simulink model "Simscape2"  (R2025b)
settings: Solver=FixedStepAuto  StartTime=0.0  StopTime=tend  FixedStep=TT_c  RelTol=1e-4  EnableMultiTasking=on
values from neighbouring files (symbols this model uses):
  alpha = 3.93e-3    (= 0.00393)    [Script_caricamento_dati_simscape2.m]
  Cr = In*2/4*Kc_act    (= 0.548435475)    [Script_caricamento_dati_simscape2.m]
  Crn = In*Kc_nom    (= 1.09116)    [Script_caricamento_dati_simscape2.m]
  f_AC_corr = [f_AC(1); f_AC(5:end)]    [Script_caricamento_dati_simscape2.m]
  In = 14    [Script_caricamento_dati_simscape2.m]
  isq0 = (B*wdq0/J + np*Cr0/J)/(Kc*np/J + ms*np^(2)*(Lsd-Lsq)*isd0/(2*J))    (= 0)    [Script_caricamento_dati_simscape2.m]
  J = 0.04e-3*3    (= 0.00012)    [Script_caricamento_dati_simscape2.m]
  kaisd = 1000    [Script_caricamento_dati_simscape2.m]
  kaisq = 1000    [Script_caricamento_dati_simscape2.m]
  kawr = 1000    [Script_caricamento_dati_simscape2.m]
  kiisd = kpisd/tiisd    (= 13158.2733813)    [Script_caricamento_dati_simscape2.m]
  kiisq = kpisq/tiisq    (= 13158.2733813)    [Script_caricamento_dati_simscape2.m]
  kiPLL = 2.5e6    (= 2500000)    [Script_caricamento_dati_simscape2.m]
  kiwr = 600    [Script_caricamento_dati_simscape2.m]
  kpisd = 23.6    [Script_caricamento_dati_simscape2.m]
  kpisq = 23.6    [Script_caricamento_dati_simscape2.m]
  kpPLL = 15    [Script_caricamento_dati_simscape2.m]
  kpwr = 0.12    [Script_caricamento_dati_simscape2.m]
  lambdam_Matrix = [1 1 1; 1 1 1; 1 1 1]    [Script_caricamento_dati_simscape2.m]
  Lsd = 1.251e-3    (= 0.001251)    [Script_caricamento_dati_simscape2.m]
  Lsd_Matrix = [1 1 1; 1 1 1; 1 1 1]    [Script_caricamento_dati_simscape2.m]
  Lsq = Lsd    (= 0.001251)    [Script_caricamento_dati_simscape2.m]
  Lsq_Matrix = [1 1 1; 1 1 1; 1 1 1]    [Script_caricamento_dati_simscape2.m]
  np = 2    [Script_caricamento_dati_simscape2.m]
  np_res = 2    [Script_caricamento_dati_simscape2.m]
  Pmax = 3*Vdc/2*Imax    (= 17010)    [Script_caricamento_dati_simscape2.m]
  Psim = 26.82e-3    (= 0.02682)    [Script_caricamento_dati_simscape2.m]
  Ratio_Rs_AC = (Rs_AC_corr-Rs)/Rs    [Script_caricamento_dati_simscape2.m]
  Rs = 0.6975    [Script_caricamento_dati_simscape2.m]
  Tmax = 1.5*Crn    (= 1.63674)    [Script_caricamento_dati_simscape2.m]
  Tphase = 100    [Script_caricamento_dati_simscape2.m]
  Trif = 298.15    [Script_caricamento_dati_simscape2.m]
  TT_c = TT_swt/100    (= 5e-07)    [Script_caricamento_dati_simscape2.m]
  TT_sc = 5e-5    (= 5e-05)    [Script_caricamento_dati_simscape2.m]
  TT_swt = 5e-5    (= 5e-05)    [Script_caricamento_dati_simscape2.m]
  Vdc = 540    [Script_caricamento_dati_simscape2.m]
  wrn = 30000    [Script_caricamento_dati_simscape2.m]
  wrr = wrn/5*1    (= 6000)    [Script_caricamento_dati_simscape2.m]
undefined symbols (not defined in the file or in its folder): denZC_id, denZC_iq, ee_sli_rtmsupport, gcbh, lambdam, numZC_id, numZC_iq
libraries: fl_lib x28, nesl_utility x22, ee_lib x14, eeTransforms x7, eeGeneralControl x6, eeDiscretePi x2, dspstat3 x1, batteryecm_lib x1, eeDqVoltageLimiter x1, eePmsmCurrentReferenceGen x1, eeVelocityController x1, eePwmGeneratorTwoLevel x1
(part 3 of 3)

== system Simscape2/PMSM Field-Oriented Control/Inner loop control ==
  idq_ref : Inport
  wElectrical : Inport  Port=2
  iabc : Inport  Port=3
  theta : Inport  Port=4
  Vdc : Inport  Port=5
  Constant : Constant  Value=0  SampleTime=-1
  Gain : Gain  Gain=1/sqrt(3)
  PMSM Current Controller with Pre-Control : Subsystem  AncestorBlock=eePmsmCurrentController/PMSM Current Controller with Pre-Control  LoadFcn=ee_sli_rtmsupport( 'loadfcn', gcbh );  mask(PMSM Current Controller with Pre-Control){Kp_id=Kp_id, Ki_id=Ki_id, Kaw_id=Kaw_id, Kp_iq=Kp_iq, Ki_iq=Ki_iq, Kaw_iq=Kaw_iq, Ts=Tsc, Tsd=0.001, AxisPrio=D-Q equivalence, ActZC=off, ActFF=on, idVect=idVect, iqVect=iqVect, LdMatrix=LdMatrix, LqMatrix=LqMatrix, psimMatrix=psimMatrix}
      mask prompts: Kp_id "physmod:ee:library:comments:control:eePmsmCurrentController:DaxisCurrentProportionalGain_MP"; Ki_id "physmod:ee:library:comments:control:eePmsmCurrentController:DaxisCurrentIntegralGain_MP"; Kaw_id "physmod:ee:library:comments:control:eePmsmCurrentController:DaxisCurrentAntiwindupGain_MP"; Kp_iq "physmod:ee:library:comments:control:eePmsmCurrentController:QaxisCurrentProportionalGain_MP"; Ki_iq "physmod:ee:library:comments:control:eePmsmCurrentController:QaxisCurrentIntegralGain_MP"; Kaw_iq "physmod:ee:library:comments:control:eePmsmCurrentController:QaxisCurrentAntiwindupGain_MP"; Ts "physmod:ee:library:comments:control:eePmsmCurrentController:SampleTime1ForInherited_MP"; Tsd "physmod:ee:library:comments:control:eePmsmCurrentController:DiscretizationSampleTime_MP"; AxisPrio "physmod:ee:library:comments:control:eePmsmCurrentController:AxisPrioritization_MP"; ActZC "physmod:ee:library:comments:control:eePmsmCurrentController:EnableZeroCancellation_MP"; ActFF "physmod:ee:library:comments:control:eePmsmCurrentController:EnablePrecontrolVoltage_MP"; idVect "physmod:ee:library:comments:control:eePmsmCurrentController:DaxisCurrentVectorIdA_MP"; iqVect "physmod:ee:library:comments:control:eePmsmCurrentController:QaxisCurrentVectorIqA_MP"; LdMatrix "physmod:ee:library:comments:control:eePmsmCurrentController:LdMatrixLdidiqH_MP"; LqMatrix "physmod:ee:library:comments:control:eePmsmCurrentController:LqMatrixLqidiqH_MP"; psimMatrix "physmod:ee:library:comments:control:eePmsmCurrentController:PermanentMagnetFluxLinkageMatrixPMidiqWb_MP"
      mask help: physmod:ee:library:comments:control:eePmsmCurrentController:PMSMCurrentControllerWithPreControl_MD
      mask init:
      | [Tsd, numZC_id, denZC_id, numZC_iq, denZC_iq] = ee.mask.initializePmsmCurrentController(ActZC,Ts,Tsd,Kp_id,Ki_id,Kp_iq,Ki_iq);
      | 
      | if length(idVect) < 2            
      | 	error(message('physmod:simscape:compiler:patterns:checks:LengthGreaterThanOrEqual',getString(message('physmod:ee:library:comments:control:eePmsmCurrentController:DaxisCurrentVectorIdA_MP')), '2'));            
      | end
      | if ~all(diff(idVect) > 0)            
      | 	error(message('physmod:simscape:compiler:patterns:checks:StrictlyAscendingVec',getString(message('physmod:ee:library:comments:control:eePmsmCurrentController:DaxisCurrentVectorIdA_MP'))));            
      | end
      | if length(iqVect) < 2            
      | 	error(message('physmod:simscape:compiler:patterns:checks:LengthGreaterThanOrEqual',getString(message('physmod:ee:library:comments:control:eePmsmCurrentController:QaxisCurrentVectorIqA_MP')), '2'));            
      | end
      | if ~all(diff(iqVect) > 0)            
      | 	error(message('physmod:simscape:compiler:patterns:checks:StrictlyAscendingVec',getString(message('physmod:ee:library:comments:control:eePmsmCurrentController:QaxisCurrentVectorIqA_MP'))));            
      | end
      | if ~all(size(LdMatrix) == [length(idVect), length(iqVect)])            
      | 	error(message('physmod:simscape:compiler:patterns:checks:Size2DEqual',getString(message('physmod:ee:library:comments:control:eePmsmCurrentController:LdMatrixLdidiqH_MP')), getString(message('physmod:ee:library:comments:control:eePmsmCurrentController:DaxisCurrentVectorIdA_MP')), getString(message('physmod:ee:library:comments:control:eePmsmCurrentController:QaxisCurrentVectorIqA_MP'))));            
      | end
      | if ~all(size(LqMatrix) == [length(idVect), length(iqVect)])            
      | 	error(message('physmod:simscape:compiler:patterns:checks:Size2DEqual',getString(message('physmod:ee:library:comments:control:eePmsmCurrentController:LqMatrixLqidiqH_MP')), getString(message('physmod:ee:library:comments:control:eePmsmCurrentController:DaxisCurrentVectorIdA_MP')), getString(message('physmod:ee:library:comments:control:eePmsmCurrentController:QaxisCurrentVectorIqA_MP'))));            
      | end
      | if ~all(size(psimMatrix) == [length(idVect), length(iqVect)])            
      | 	error(message('physmod:simscape:compiler:patterns:checks:Size2DEqual',getString(message('physmod:ee:library:comments:control:eePmsmCurrentController:PermanentMagnetFluxLinkageMatrixPMidiqWb_MP')), getString(message('physmod:ee:library:comments:control:eePmsmCurrentController:DaxisCurrentVectorIdA_MP')), getString(message('physmod:ee:library:comments:control:eePmsmCurrentController:QaxisCurrentVectorIqA_MP'))));            
      | end
      settings: CopyFcn=ee_sli_rtmsupport( 'copyfcn', gcbh );  DeleteFcn=ee_sli_rtmsupport( 'deletefcn', gcbh );  ModelCloseFcn=ee_sli_rtmsupport( 'modelclosefcn', gcbh );  PostSaveFcn=ee_sli_rtmsupport( 'postsavefcn', gcbh );  PreCopyFcn=ee_sli_rtmsupport( 'precopyfcn', gcbh );  OpenFcn=ee_sli_rtmsupport( 'openfcn', gcbh );  CloseFcn=ee_sli_rtmsupport( 'closefcn', gcbh );  PreDeleteFcn=ee_sli_rtmsupport( 'predeletefcn', gcbh );
      mask Help: web(nesl_help(gcbh))
      mask Callback Ts: ee.mask.callbackZeroCancellation(gcb);
      mask TypeOptions AxisPrio: d-q Voltage Limiter/AxisPrio
      mask Callback ActZC: ee.mask.callbackZeroCancellation(gcb);
      mask DialogControl Container3 Prompt: physmod:ee:library:comments:control:eePmsmCurrentController:tab_ControlParameters
      mask DialogControl Kp_id Prompt: D-axis current proportional gain
      mask DialogControl Ki_id Prompt: D-axis current integral gain
      mask DialogControl Kaw_id Prompt: D-axis current anti-windup gain
      mask DialogControl Kp_iq Prompt: Q-axis current proportional gain
      mask DialogControl Ki_iq Prompt: Q-axis current integral gain
      mask DialogControl Kaw_iq Prompt: Q-axis current anti-windup gain
      mask DialogControl Ts Prompt: Sample time (-1 for inherited)
      mask DialogControl Tsd Prompt: Discretization sample time
      mask DialogControl AxisPrio Prompt: Axis prioritization
      mask DialogControl ActZC Prompt: Enable zero cancellation
      mask DialogControl ActFF Prompt: Enable pre-control voltage
      mask DialogControl Container4 Prompt: physmod:ee:library:comments:control:eePmsmCurrentController:tab_PreControlParameters
      mask DialogControl idVect Prompt: D-axis current vector, id (A)
      mask DialogControl iqVect Prompt: Q-axis current vector, iq (A)
      mask DialogControl LdMatrix Prompt: Ld matrix, Ld(id,iq), (H)
      mask DialogControl LqMatrix Prompt: Lq matrix, Lq(id,iq), (H)
      mask DialogControl psimMatrix Prompt: Permanent magnet flux linkage matrix, PM(id,iq), (Wb)
  Park Transform : eeTransforms/Park Transform  AxisAlignment=D-axis  PowerInvariant=off
  Selector : Selector  InputPortWidth=3  IndexOptions=Index vector (dialog)  Indices=[1 2]  OutputSizes=1
  vdqRef : Outport  VectorParamsAs1DForOutWhenUnconnected=off
  idq : Outport  Port=2  VectorParamsAs1DForOutWhenUnconnected=off
  wires:
  PMSM Current Controller with Pre-Control/1(vdqRef) -> vdqRef/1
  Vdc/1 -> Gain/1
  wElectrical/1 -> PMSM Current Controller with Pre-Control/3(wElectrical)
  theta/1 -> Park Transform/2
  iabc/1 -> Park Transform/1
  idq_ref/1 -> PMSM Current Controller with Pre-Control/1(idqRef)
  Park Transform/1 -> Selector/1
  Gain/1 -> PMSM Current Controller with Pre-Control/4(VphMax)
  Selector/1 -> idq/1, PMSM Current Controller with Pre-Control/2(idq)
  Constant/1 -> PMSM Current Controller with Pre-Control/5(Reset)

== system Simscape2/PMSM Field-Oriented Control/Input interface ==
  iabcSens : Inport
  wSens : Inport  Port=2
  thSens : Inport  Port=3
  VdcSens : Inport  Port=4
  2*pi : Constant  Value=2*pi  SampleTime=Tsc
  Math Function : Math  Operator=mod  SignedPower=on
  Relay : Relay  OnSwitchValue=Vdc_on  OffSwitchValue=0.5*Vdc_on
  pole pairs : Gain  Gain=p
  "pole pairs " : Gain  Gain=p
  wElectrical : Outport  VectorParamsAs1DForOutWhenUnconnected=off
  iabc : Outport  Port=2  VectorParamsAs1DForOutWhenUnconnected=off
  theta : Outport  Port=3  VectorParamsAs1DForOutWhenUnconnected=off
  Vdc : Outport  Port=4  VectorParamsAs1DForOutWhenUnconnected=off
  PwmEnable : Outport  Port=5  VectorParamsAs1DForOutWhenUnconnected=off
  wires:
  VdcSens/1 -> Vdc/1, Relay/1
  Relay/1 -> PwmEnable/1
  Math Function/1 -> theta/1
  2*pi/1 -> Math Function/2
  "pole pairs "/1 -> Math Function/1
  iabcSens/1 -> iabc/1
  wSens/1 -> pole pairs/1
  thSens/1 -> "pole pairs "/1
  pole pairs/1 -> wElectrical/1

== system Simscape2/PMSM Field-Oriented Control/Outer loop control ==
  Reference : Inport
  wElectrical : Inport  Port=2
  Vdc : Inport  Port=3
  Constant : Constant  Value=0  SampleTime=-1
  PMSM Current Reference Generator : eePmsmCurrentReferenceGen/PMSM Current Reference Generator  Vnom=Vnom  Pmax=Pmax  Tmax=Tmax  Ts=Tsc  RefType=Zero d-axis control  rpmVec=rpmVec  TqVec=TqVec  VdcVec=VdcVec  PWMMode=SPWM: sinusoidal PWM  ModFactor=ModFactor  idMatrix=idMatrix  iqMatrix=iqMatrix  p=p  psim=psim  Ld=Ld  Lq=Lq  Rs=Rs  RefExpEnable=0
      link override idRef: Value=0
  Tq Selector : Subsystem
  Velocity Controller : eeVelocityController/Velocity Controller  CtrlType=PI control  Kp_w=Kp_w  Ki_w=Ki_w  Kv_w=Kv_w  Kaw_w=Kaw_w  Ts=Tsc  Tsd=0.001  ActZC=off
  elec->mech : Gain  Gain=1/p
  idqRef : Outport  VectorParamsAs1DForOutWhenUnconnected=off
  TqRef : Outport  Port=2  VectorParamsAs1DForOutWhenUnconnected=off
  TqLim : Outport  Port=3  VectorParamsAs1DForOutWhenUnconnected=off
  wires:
  Velocity Controller/1 -> Tq Selector/2(TqRefUnsat)
  Tq Selector/1(TqRef) -> PMSM Current Reference Generator/1
  Constant/1 -> Velocity Controller/4
  elec->mech/1 -> Velocity Controller/2, PMSM Current Reference Generator/2
  PMSM Current Reference Generator/3 -> TqLim/1
  PMSM Current Reference Generator/2 -> TqRef/1, Velocity Controller/3
  PMSM Current Reference Generator/1 -> idqRef/1
  Vdc/1 -> PMSM Current Reference Generator/3
  wElectrical/1 -> elec->mech/1
  Reference/1 -> Tq Selector/1(Reference), Velocity Controller/1

== system Simscape2/PMSM Field-Oriented Control/PWM ==
  vdqRef : Inport
  theta : Inport  Port=2
  Vdc : Inport  Port=3
  PwmEnable : Inport  Port=4
  Constant : Constant  Value=0  SampleTime=Tsc
  Inverse Park Transform : eeTransforms/Inverse Park Transform  AxisAlignment=D-axis  PowerInvariant=off
  Mux : Mux  Inputs=2
  "PWM Generator (Three-phase, Two-level)" : eePwmGeneratorTwoLevel/PWM Generator (Three-phase, Two-level)  PWMMode=Continuous PWM (CPWM)  CPWMMode=SPWM: sinusoidal PWM  DPWMMode=60 DPWM: 60 degree discontinuous PWM  fsw=fsw  Ts=Ts
      settings: SamplingMode=Symmetric
  Switch1 : Switch  Criteria=u2 > Threshold  SaturateOnIntegerOverflow=off  InputSameDT=off
  To Workspace : ToWorkspace  VariableName=Vabc_ref  SampleTime=-1
  Unit Delay2 : UnitDelay  SampleTime=Tsc  HasFrameUpgradeWarning=on
  Zero vector : Constant  Value=zeros(6,1)  SampleTime=Ts
  G : Outport  VectorParamsAs1DForOutWhenUnconnected=off
  ModWave : Outport  Port=2  SampleTime=Tsc  VectorParamsAs1DForOutWhenUnconnected=off
  wires:
  Unit Delay2/1 -> Switch1/2
  Vdc/1 -> "PWM Generator (Three-phase, Two-level)"/2
  Inverse Park Transform/1 -> To Workspace/1, "PWM Generator (Three-phase, Two-level)"/1
  Switch1/1 -> G/1
  Zero vector/1 -> Switch1/3
  PwmEnable/1 -> Unit Delay2/1
  "PWM Generator (Three-phase, Two-level)"/1 -> Switch1/1
  "PWM Generator (Three-phase, Two-level)"/2 -> ModWave/1
  Constant/1 -> Mux/2
  Mux/1 -> Inverse Park Transform/1
  vdqRef/1 -> Mux/1
  theta/1 -> Inverse Park Transform/2

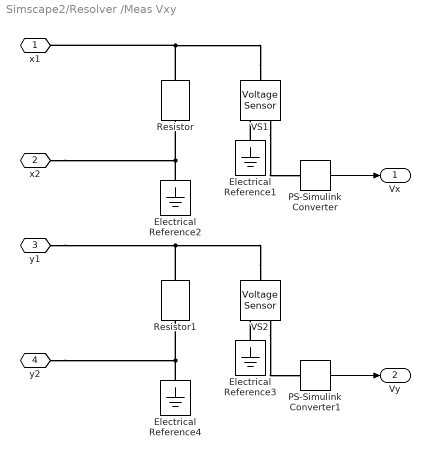
== system Simscape2/Resolver /Meas Vxy ==
  Electrical Reference{1..4} (4 alike) : fl_lib/Electrical/Electrical Elements/Electrical Reference
  PS-Simulink Converter : nesl_utility/PS-Simulink Converter  PhysicalDomain=network_engine_domain  SubClassName=ps_output  LeftPortType=input  RightPortType=output  PseudoPeriodic=off  Frequencies=[]  Unit=1  AffineConversion=off
  PS-Simulink Converter1 : nesl_utility/PS-Simulink Converter  PhysicalDomain=network_engine_domain  SubClassName=ps_output  LeftPortType=input  RightPortType=output  PseudoPeriodic=off  Frequencies=[]  Unit=1  AffineConversion=off
  Resistor : fl_lib/Electrical/Electrical Elements/Resistor  R=1e3 Ohm  i_specify=off  i_priority=None  i=0 A  i_nominal_specify=off  i_nominal_unit=A  i_nominal_value=1  v_specify=off  v_priority=None  v=0 V  v_nominal_specify=off  v_nominal_unit=V  v_nominal_value=1
  Resistor1 : fl_lib/Electrical/Electrical Elements/Resistor  R=1e3 Ohm  i_specify=off  i_priority=None  i=0 A  i_nominal_specify=off  i_nominal_unit=A  i_nominal_value=1  v_specify=off  v_priority=None  v=0 V  v_nominal_specify=off  v_nominal_unit=V  v_nominal_value=1
  VS1 : fl_lib/Electrical/Electrical Sensors/Voltage Sensor
  VS2 : fl_lib/Electrical/Electrical Sensors/Voltage Sensor
  x1 : PMIOPort  Side=Left
  x2 : PMIOPort  Port=2  Side=Left
  y1 : PMIOPort  Port=3  Side=Left
  y2 : PMIOPort  Port=4  Side=Left
  Vx : Outport
  Vy : Outport  Port=2
  wires:
  PS-Simulink Converter/1 -> Vx/1
  PS-Simulink Converter1/1 -> Vy/1
  connections:
  VS1/LConn1 -- x1/RConn1 -- Resistor/LConn1
  VS1/RConn1 -- PS-Simulink Converter/LConn1
  Resistor/RConn1 -- x2/RConn1 -- Electrical Reference2/LConn1
  Electrical Reference1/LConn1 -- VS1/RConn2
  y2/RConn1 -- Electrical Reference4/LConn1 -- Resistor1/RConn1
  VS2/LConn1 -- y1/RConn1 -- Resistor1/LConn1
  Electrical Reference3/LConn1 -- VS2/RConn2
  VS2/RConn1 -- PS-Simulink Converter1/LConn1

== system Simscape2/Resolver /Vp ==
  Electrical Reference1 : fl_lib/Electrical/Electrical Elements/Electrical Reference
  PS-Simulink Converter2 : nesl_utility/PS-Simulink Converter  PhysicalDomain=network_engine_domain  SubClassName=ps_output  LeftPortType=input  RightPortType=output  PseudoPeriodic=off  Frequencies=[]  Unit=1  AffineConversion=off
  VS1 : fl_lib/Electrical/Electrical Sensors/Voltage Sensor
  Vp1 : fl_lib/Electrical/Electrical Sources/AC Voltage Source  amp=5 V  shift=0 rad  frequency=1e4 Hz  omega=0 rad/s
  p1 : PMIOPort  Side=Right
  p2 : PMIOPort  Port=2  Side=Right
  Vp : Outport
  wires:
  PS-Simulink Converter2/1 -> Vp/1
  connections:
  VS1/RConn1 -- PS-Simulink Converter2/LConn1
  Electrical Reference1/LConn1 -- p2/RConn1 -- VS1/RConn2 -- Vp1/RConn1
  VS1/LConn1 -- Vp1/LConn1 -- p1/RConn1

== system Simscape2/Sensing currents1/LEM current sensor uncertainty ==
  In1 : Inport
  Demux : Demux  Outputs=3
  Mux : Mux  Inputs=3
  Offset : Constant  Value=0
  Offset1 : Constant  Value=0
  Offset2 : Constant  Value=0
  Product : Product
  Product2 : Product
  Product3 : Product
  Sum : Sum  Inputs=|++
  Sum1 : Sum  Inputs=|++
  Sum2 : Sum  Inputs=|++
  Uniform Random Number : UniformRandomNumber  Minimum=-0.0065  Maximum=0.0065  SampleTime=TT_c
  Out1 : Outport
  wires:
  Product/1 -> Sum/2
  Sum1/1 -> Mux/2
  Uniform Random Number/1 -> Product3/2, Product2/2, Product/2
  In1/1 -> Demux/1
  Offset/1 -> Sum/1
  Sum2/1 -> Mux/3
  Sum/1 -> Mux/1
  Mux/1 -> Out1/1
  Demux/1 -> Product/1
  Product3/1 -> Sum2/2
  Product2/1 -> Sum1/2
  Demux/3 -> Product3/1
  Demux/2 -> Product2/1
  Offset1/1 -> Sum1/1
  Offset2/1 -> Sum2/1

== system Simscape2/Three-phase inverter/LEM voltage sensor uncertainty ==
  In1 : Inport
  Product : Product
  Uniform Random Number : UniformRandomNumber  Minimum=-0.008  Maximum=0.008  SampleTime=TT_c
  Out1 : Outport
  wires:
  Uniform Random Number/1 -> Product/2
  In1/1 -> Product/1
  Product/1 -> Out1/1

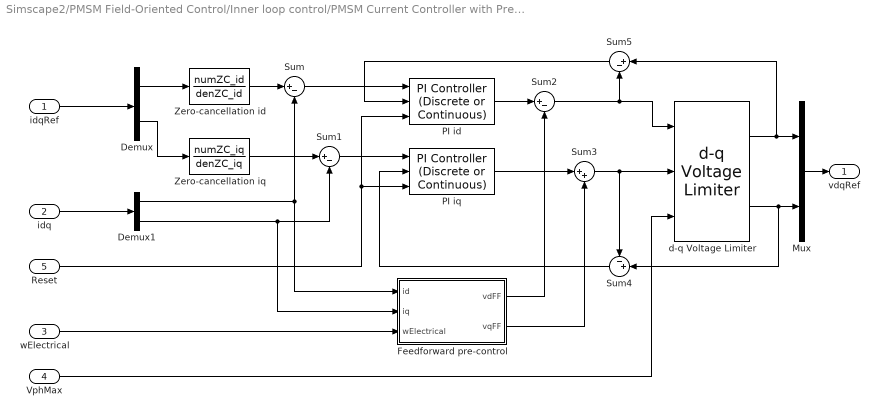
== system Simscape2/PMSM Field-Oriented Control/Inner loop control/PMSM Current Controller with Pre-Control ==
  idqRef : Inport  SampleTime=Ts
  idq : Inport  Port=2  SampleTime=Ts
  wElectrical : Inport  Port=3  SampleTime=Ts
  VphMax : Inport  Port=4  SampleTime=Ts
  Reset : Inport  Port=5  SampleTime=Ts
  Demux : Demux  Outputs=2
  Demux1 : Demux  Outputs=2
  Feedforward pre-control : Subsystem
  Mux : Mux  Inputs=2
  PI id : eeDiscretePi/PI Controller (Discrete or Continuous)  Kp=Kp_id  Ki=Ki_id  Kaw=Kaw_id  x0=0  Ts=Ts
  PI iq : eeDiscretePi/PI Controller (Discrete or Continuous)  Kp=Kp_iq  Ki=Ki_iq  Kaw=Kaw_iq  x0=0  Ts=Ts
  Sum{,1..2,5} (4 alike) : Sum  Inputs=|+-
  Sum3 : Sum  Inputs=|++
  Sum4 : Sum  Inputs=-+|
  Zero-cancellation id : DiscreteTransferFcn  Numerator=numZC_id  Denominator=denZC_id  SampleTime=Ts
  Zero-cancellation iq : DiscreteTransferFcn  Numerator=numZC_iq  Denominator=denZC_iq  SampleTime=Ts
  d-q Voltage Limiter : eeDqVoltageLimiter/d-q Voltage Limiter  AxisPrio=D-Q equivalence  Ts=Ts
  vdqRef : Outport  VectorParamsAs1DForOutWhenUnconnected=off
  wires:
  VphMax/1 -> d-q Voltage Limiter/3
  wElectrical/1 -> Feedforward pre-control/3(wElectrical)
  Reset/1 -> PI id/3, PI iq/3
  idq/1 -> Demux1/1
  idqRef/1 -> Demux/1
  Sum5/1 -> PI id/2
  Demux1/2 -> Sum1/2, Feedforward pre-control/2(iq)
  Demux1/1 -> Sum/2, Feedforward pre-control/1(id)
  d-q Voltage Limiter/2 -> Sum4/2, Mux/2
  Sum4/1 -> PI iq/2
  Feedforward pre-control/2(vqFF) -> Sum3/2
  Demux/2 -> Zero-cancellation iq/1
  Sum3/1 -> Sum4/1, d-q Voltage Limiter/2
  Demux/1 -> Zero-cancellation id/1
  d-q Voltage Limiter/1 -> Sum5/1, Mux/1
  Sum/1 -> PI id/1
  Sum1/1 -> PI iq/1
  PI id/1 -> Sum2/1
  Zero-cancellation iq/1 -> Sum1/1
  PI iq/1 -> Sum3/1
  Mux/1 -> vdqRef/1
  Zero-cancellation id/1 -> Sum/1
  Sum2/1 -> Sum5/2, d-q Voltage Limiter/1
  Feedforward pre-control/1(vdFF) -> Sum2/2

== system Simscape2/PMSM Field-Oriented Control/Outer loop control/Tq Selector ==
  Reference : Inport
  TqRefUnsat : Inport  Port=2
  Constant : Constant  Value=CtrlMode  SampleTime=Tsc
  Switch : Switch  Criteria=u2 > Threshold  Threshold=1.5  SaturateOnIntegerOverflow=off  InputSameDT=off
  TqRef : Outport  VectorParamsAs1DForOutWhenUnconnected=off
  wires:
  Switch/1 -> TqRef/1
  Constant/1 -> Switch/2
  TqRefUnsat/1 -> Switch/3
  Reference/1 -> Switch/1

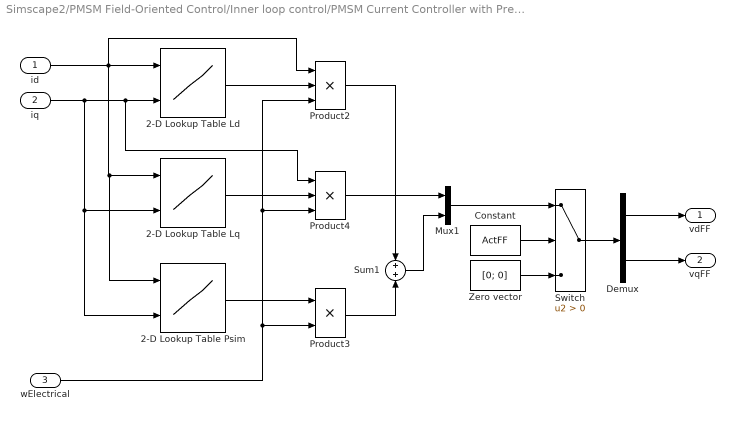
== system Simscape2/PMSM Field-Oriented Control/Inner loop control/PMSM Current Controller with Pre-Control/Feedforward pre-control ==
  id : Inport
  iq : Inport  Port=2
  wElectrical : Inport  Port=3
  2-D Lookup Table Ld : Lookup_n-D  BreakpointsForDimension1=idVect  BreakpointsForDimension2=iqVect  Table=LdMatrix  ExtrapMethod=Clip  UseLastTableValue=on  InternalRulePriority=Speed  RndMeth=Simplest
      settings: InputPortMap=u0,u1
  2-D Lookup Table Lq : Lookup_n-D  BreakpointsForDimension1=idVect  BreakpointsForDimension2=iqVect  Table=LqMatrix  ExtrapMethod=Clip  InternalRulePriority=Speed  RndMeth=Simplest
      settings: InputPortMap=u0,u1
  2-D Lookup Table Psim : Lookup_n-D  BreakpointsForDimension1=idVect  BreakpointsForDimension2=iqVect  Table=psimMatrix  ExtrapMethod=Clip  InternalRulePriority=Speed  RndMeth=Simplest
      settings: InputPortMap=u0,u1
  Constant : Constant  Value=ActFF  SampleTime=Ts
  Demux : Demux  Outputs=2
  Mux1 : Mux  Inputs=2
  Product2 : Product  Inputs=3
  Product3 : Product
  Product4 : Product  Inputs=3
  Sum1 : Sum
  Switch : Switch  Criteria=u2 > Threshold  SaturateOnIntegerOverflow=off  InputSameDT=off
  Zero vector : Constant  Value=[0; 0]  SampleTime=Ts
  vdFF : Outport  VectorParamsAs1DForOutWhenUnconnected=off
  vqFF : Outport  Port=2  VectorParamsAs1DForOutWhenUnconnected=off
  wires:
  Product2/1 -> Sum1/1
  wElectrical/1 -> Product2/3, Product4/3, Product3/2
  Mux1/1 -> Switch/1
  Product4/1 -> Mux1/1
  id/1 -> 2-D Lookup Table Ld/1, 2-D Lookup Table Lq/1, 2-D Lookup Table Psim/1, Product2/1
  iq/1 -> 2-D Lookup Table Psim/2, 2-D Lookup Table Lq/2, 2-D Lookup Table Ld/2, Product4/1
  2-D Lookup Table Ld/1 -> Product2/2
  Sum1/1 -> Mux1/2
  Zero vector/1 -> Switch/3
  2-D Lookup Table Psim/1 -> Product3/1
  Demux/2 -> vqFF/1
  Demux/1 -> vdFF/1
  Switch/1 -> Demux/1
  Constant/1 -> Switch/2
  2-D Lookup Table Lq/1 -> Product4/2
  Product3/1 -> Sum1/2
